simulink subsystem "icub_head"  (R2024a)
settings: Solver=VariableStepAuto  StartTime=0.0  StopTime=10.0  RelTol=1e-3
undefined symbols (not defined in the file): headData, iCubHeadData, X, Y, Z
libraries: sm_lib x7
settings Model: DataDictionary=icub_head_data.sldd  EnableAccessToBaseWorkspace=off  Creator=ngenesio  LastModifiedBy=upattacini
settings RTWCC: GPUComputeCapability=3.5

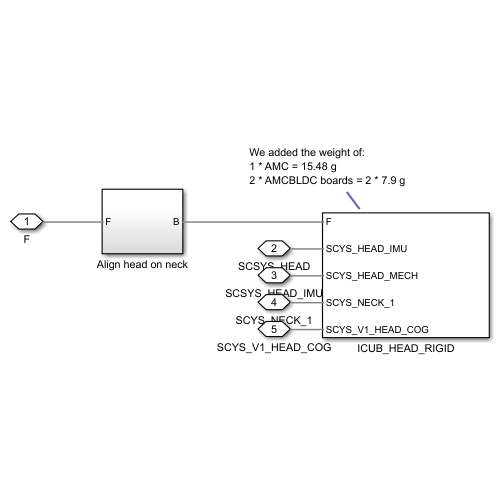
[thumbnail: Simulink's stored preview of the top-level diagram]
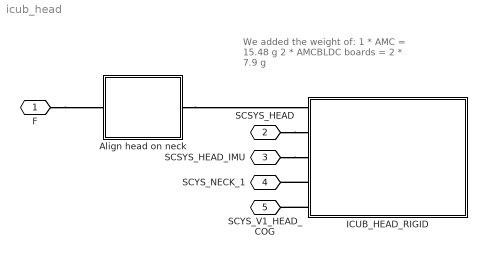
== system icub_head ==
  note: We added the weight of:
      | 1 * AMC = 15.48 g
      | 2 * AMCBLDC boards = 2 * 7.9 g
  Align head on neck : Subsystem
  ICUB_HEAD_RIGID : Subsystem
  F : PMIOPort  Side=Left
  SCSYS_HEAD : PMIOPort  Port=2  Side=Left
  SCSYS_HEAD_IMU : PMIOPort  Port=3  Side=Left
  SCYS_NECK_1 : PMIOPort  Port=4  Side=Left
  SCYS_V1_HEAD_COG : PMIOPort  Port=5  Side=Left
  connections:
  ICUB_HEAD_RIGID/LConn5 -- SCYS_V1_HEAD_COG/RConn1
  F/RConn1 -- Align head on neck/RConn1
  SCSYS_HEAD_IMU/RConn1 -- ICUB_HEAD_RIGID/LConn3
  Align head on neck/LConn1 -- ICUB_HEAD_RIGID/LConn1
  SCSYS_HEAD/RConn1 -- ICUB_HEAD_RIGID/LConn2
  ICUB_HEAD_RIGID/LConn4 -- SCYS_NECK_1/RConn1

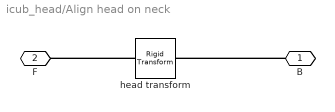
== system icub_head/Align head on neck ==
  head transform : sm_lib/Frames and Transforms/Rigid Transform  RotationMethod=RotationSequence  FollAlignAxisA=+X  BaseAlignAxisA=+Y  FollAlignAxisB=+Y  BaseAlignAxisB=+Z  RotationStandardAxis=+Z  RotationAngle=headData.RigidTransform(4).angle  RotationAngleUnits=rad  RotationArbitraryAxis=headData.RigidTransform(4).axis  RotationSequenceAxes=FollowerAxes  RotationSequence=XYX  RotationSequenceAngles=[0 90 0]  RotationSequenceAnglesUnits=deg  RotationMatrix=[1 0 0; 0 1 0; 0 0 1]  Quaternion=[1 0 0 0]  TranslationMethod=Cartesian  TranslationCartesianOffset=[21.05 -7.7 0]  TranslationCartesianOffsetUnits=mm  TranslationStandardAxis=+Z  TranslationStandardOffset=0  TranslationStandardOffsetUnits=mm  TranslationROffset=0  TranslationROffsetUnits=m  TranslationThetaOffset=0  TranslationThetaOffsetUnits=deg  TranslationZOffset=0  TranslationZOffsetUnits=m
  B : PMIOPort  Side=Left
  F : PMIOPort  Port=2  Side=Right
  connections:
  head transform/LConn1 -- F/RConn1
  B/RConn1 -- head transform/RConn1

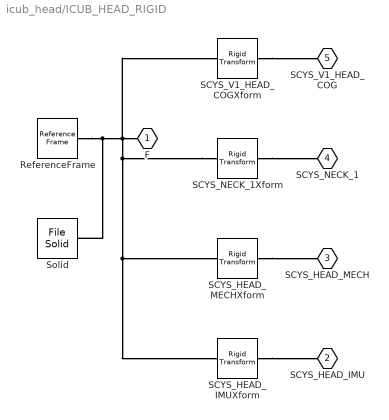
== system icub_head/ICUB_HEAD_RIGID ==
  ReferenceFrame : sm_lib/Frames and Transforms/Reference Frame
  SCYS_HEAD_IMUXform : sm_lib/Frames and Transforms/Rigid Transform  RotationMethod=ArbitraryAxis  FollAlignAxisA=+X  BaseAlignAxisA=+Y  FollAlignAxisB=+Y  BaseAlignAxisB=+Z  RotationStandardAxis=+Z  RotationAngle=iCubHeadData.RigidTransform(2).angle  RotationAngleUnits=rad  RotationArbitraryAxis=iCubHeadData.RigidTransform(2).axis  RotationSequenceAxes=FollowerAxes  RotationSequence=XYX  RotationSequenceAngles=[0 0 0]  RotationSequenceAnglesUnits=deg  RotationMatrix=[1 0 0; 0 1 0; 0 0 1]  Quaternion=[1 0 0 0]  TranslationMethod=Cartesian  TranslationCartesianOffset=iCubHeadData.RigidTransform(2).translation  TranslationCartesianOffsetUnits=mm  TranslationStandardAxis=+Z  TranslationStandardOffset=0  TranslationStandardOffsetUnits=m  TranslationROffset=0  TranslationROffsetUnits=m  TranslationThetaOffset=0  TranslationThetaOffsetUnits=deg  TranslationZOffset=0  TranslationZOffsetUnits=m
  SCYS_HEAD_MECHXform : sm_lib/Frames and Transforms/Rigid Transform  RotationMethod=ArbitraryAxis  FollAlignAxisA=+X  BaseAlignAxisA=+Y  FollAlignAxisB=+Y  BaseAlignAxisB=+Z  RotationStandardAxis=+Z  RotationAngle=iCubHeadData.RigidTransform(4).angle  RotationAngleUnits=rad  RotationArbitraryAxis=iCubHeadData.RigidTransform(4).axis  RotationSequenceAxes=FollowerAxes  RotationSequence=XYX  RotationSequenceAngles=[0 0 0]  RotationSequenceAnglesUnits=deg  RotationMatrix=[1 0 0; 0 1 0; 0 0 1]  Quaternion=[1 0 0 0]  TranslationMethod=Cartesian  TranslationCartesianOffset=iCubHeadData.RigidTransform(4).translation  TranslationCartesianOffsetUnits=mm  TranslationStandardAxis=+Z  TranslationStandardOffset=0  TranslationStandardOffsetUnits=m  TranslationROffset=0  TranslationROffsetUnits=m  TranslationThetaOffset=0  TranslationThetaOffsetUnits=deg  TranslationZOffset=0  TranslationZOffsetUnits=m
  SCYS_NECK_1Xform : sm_lib/Frames and Transforms/Rigid Transform  RotationMethod=ArbitraryAxis  FollAlignAxisA=+X  BaseAlignAxisA=+Y  FollAlignAxisB=+Y  BaseAlignAxisB=+Z  RotationStandardAxis=+Z  RotationAngle=iCubHeadData.RigidTransform(3).angle  RotationAngleUnits=rad  RotationArbitraryAxis=iCubHeadData.RigidTransform(3).axis  RotationSequenceAxes=FollowerAxes  RotationSequence=XYX  RotationSequenceAngles=[0 0 0]  RotationSequenceAnglesUnits=deg  RotationMatrix=[1 0 0; 0 1 0; 0 0 1]  Quaternion=[1 0 0 0]  TranslationMethod=Cartesian  TranslationCartesianOffset=iCubHeadData.RigidTransform(3).translation  TranslationCartesianOffsetUnits=mm  TranslationStandardAxis=+Z  TranslationStandardOffset=0  TranslationStandardOffsetUnits=m  TranslationROffset=0  TranslationROffsetUnits=m  TranslationThetaOffset=0  TranslationThetaOffsetUnits=deg  TranslationZOffset=0  TranslationZOffsetUnits=m
  SCYS_V1_HEAD_COGXform : sm_lib/Frames and Transforms/Rigid Transform  RotationMethod=ArbitraryAxis  FollAlignAxisA=+X  BaseAlignAxisA=+Y  FollAlignAxisB=+Y  BaseAlignAxisB=+Z  RotationStandardAxis=+Z  RotationAngle=iCubHeadData.RigidTransform(1).angle  RotationAngleUnits=rad  RotationArbitraryAxis=iCubHeadData.RigidTransform(1).axis  RotationSequenceAxes=FollowerAxes  RotationSequence=XYX  RotationSequenceAngles=[0 0 0]  RotationSequenceAnglesUnits=deg  RotationMatrix=[1 0 0; 0 1 0; 0 0 1]  Quaternion=[1 0 0 0]  TranslationMethod=Cartesian  TranslationCartesianOffset=iCubHeadData.RigidTransform(1).translation  TranslationCartesianOffsetUnits=mm  TranslationStandardAxis=+Z  TranslationStandardOffset=0  TranslationStandardOffsetUnits=m  TranslationROffset=0  TranslationROffsetUnits=m  TranslationThetaOffset=0  TranslationThetaOffsetUnits=deg  TranslationZOffset=0  TranslationZOffsetUnits=m
  Solid : sm_lib/Body Elements/File Solid  ExtGeomFileName=icub_head_prt.step  UnitType=FromFile  ExtGeomFileUnits=m  StepReaderType=HEX  ExportConvexHullGeometry=off  InertiaType=Custom  BasedOnType=DensityFromFile  Density=1000  DensityUnits=kg/m^3  Mass=iCubHeadData.Solid(1).mass  MassUnits=kg  CenterOfMass=iCubHeadData.Solid(1).CoM  CenterOfMassUnits=mm  MomentsOfInertia=iCubHeadData.Solid(1).MoI  MomentsOfInertiaUnits=kg*mm^2  ProductsOfInertia=iCubHeadData.Solid(1).PoI  ProductsOfInertiaUnits=kg*mm^2  GraphicType=FromGeometry  MarkerShape=Sphere  MarkerSize=10  GraphicVisPropType=SimpleVisualProperties  GraphicDiffuseColor=iCubHeadData.Solid(1).color  GraphicOpacity=iCubHeadData.Solid(1).opacity  GraphicSpecularColor=[0.5 0.5 0.5 1.0]  GraphicAmbientColor=[0.15 0.15 0.15 1.0]  GraphicEmissiveColor=[0.0 0.0 0.0 1.0]  GraphicShininess=75  DoExposeReferenceFrame=on  SerializedFrames=<Frames/>
  F : PMIOPort  Side=Left
  SCYS_HEAD_IMU : PMIOPort  Port=2  Side=Left
  SCYS_HEAD_MECH : PMIOPort  Port=3  Side=Left
  SCYS_NECK_1 : PMIOPort  Port=4  Side=Left
  SCYS_V1_HEAD_COG : PMIOPort  Port=5  Side=Left
  connections:
  SCYS_HEAD_MECHXform/RConn1 -- SCYS_HEAD_MECH/RConn1
  SCYS_NECK_1Xform/RConn1 -- SCYS_NECK_1/RConn1
  SCYS_HEAD_IMUXform/RConn1 -- SCYS_HEAD_IMU/RConn1
  SCYS_V1_HEAD_COGXform/RConn1 -- SCYS_V1_HEAD_COG/RConn1
  SCYS_NECK_1Xform/LConn1 -- F/RConn1 -- SCYS_V1_HEAD_COGXform/LConn1 -- Solid/RConn1 -- ReferenceFrame/RConn1 -- SCYS_HEAD_MECHXform/LConn1 -- SCYS_HEAD_IMUXform/LConn1
